simulink model "VOO_3K04"  (R2022a)
settings: Solver=FixedStepAuto  StartTime=0.0  StopTime=10.0  FixedStep=1e-3  RelTol=1e-3  EnableMultiTasking=on
undefined symbols (not defined in the file): D10, D11, D12, D2, D4, D5, D7, D8, D9, PTA0, PTA2, PTB23, PTB9, PTC3, PTC4, PTD0, PTD2, PTD3
libraries: frdmk64flib x11
settings Model: ExtModeTrigDuration=5  Creator=patri  LastModifiedBy=joshb
settings OptimizationCC: EnhancedBackFolding=on  PassReuseOutputArgsAs=Individual arguments  ZeroExternalMemoryAtStartup=off  ZeroInternalMemoryAtStartup=off  MaxStackSize=64  OptimizeBlockOrder=speed  DifferentSizesBufferReuse=on  OptimizationCustomize=off  EfficientTunableParamExpr=on
settings DebuggingCC: ParameterTunabilityLossMsg=error
settings HardwareCC: ProdBitPerPointer=32  ProdBitPerSizeT=32  ProdBitPerPtrDiffT=32  ProdLargestAtomicInteger=Long  ProdLargestAtomicFloat=Double  ProdWordSize=32  ProdHWDeviceType=ARM Compatible->ARM Cortex
settings SFSimCC: MATLABDynamicMemAlloc=off
settings RTWCC: SystemTargetFile=ert.tlc  HardwareBoard=NXP FRDM-K64F  TLCOptions="-aInlineSetEventsForThisBaseRateFcn=TLC_FALSE -aSuppressMultiTaskScheduler=TLC_FALSE  -aRateBasedStepFcn=0"  TemplateMakefile=ert_default_tmf  Toolchain=GNU Tools for ARM Embedded Processors
settings CodeAppCC: ForceParamTrailComments=on  IgnoreCustomStorageClasses=off  OperatorAnnotations=on  SimulinkDataObjDesc=on  SFDataObjDesc=on  InsertBlockDesc=on
settings ERTTargetCC: ExtModeTransport=4  ExtModeMexFile=sendToCommService

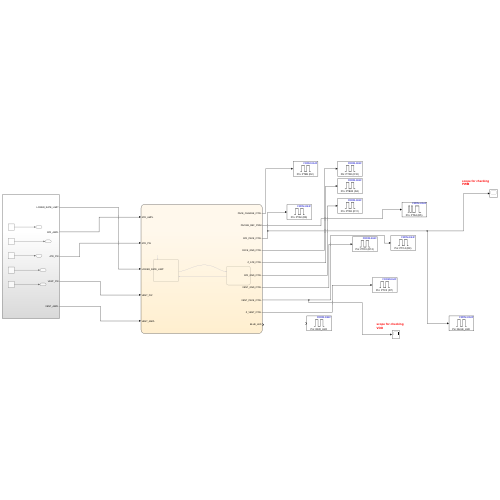
[thumbnail: Simulink's stored preview of the top-level diagram]
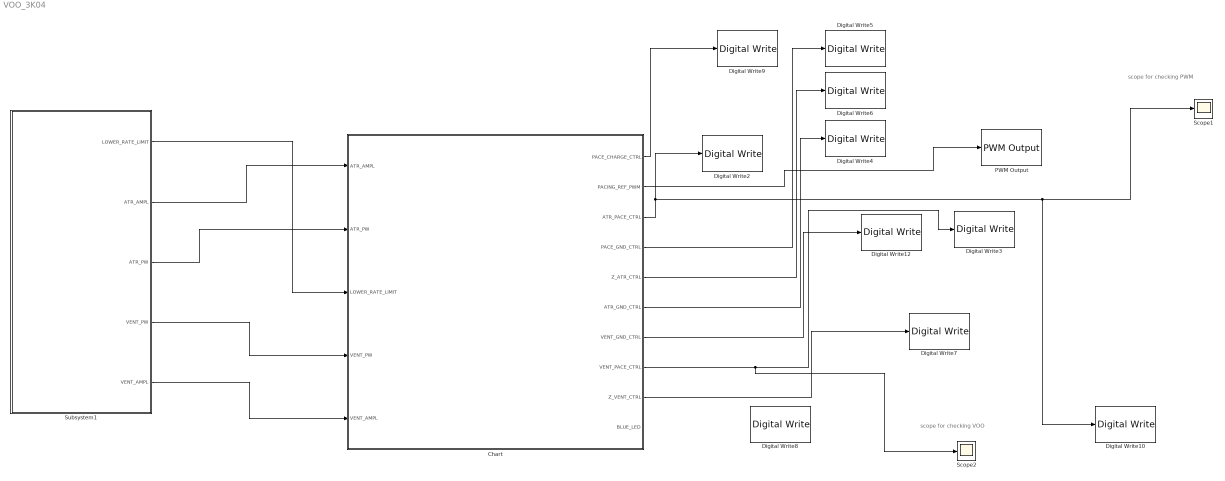
== system VOO_3K04 ==
  note: scope for checking PWM
  note: scope for checking VOO
  Chart : Stateflow chart  TreatAsAtomicUnit=on
  Digital Write10 : frdmk64flib/Digital Write  Whichpin=BLUE_LED
  Digital Write12 : frdmk64flib/Digital Write  Whichpin=PTD3 (D12)
  Digital Write2 : frdmk64flib/Digital Write  Whichpin=PTA0 (D8)
  Digital Write3 : frdmk64flib/Digital Write  Whichpin=PTC4 (D9)
  Digital Write4 : frdmk64flib/Digital Write  Whichpin=PTD2 (D11)
  Digital Write5 : frdmk64flib/Digital Write  Whichpin=PTD0 (D10)
  Digital Write6 : frdmk64flib/Digital Write  Whichpin=PTB23 (D4)
  Digital Write7 : frdmk64flib/Digital Write  Whichpin=PTC3 (D7)
  Digital Write8 : frdmk64flib/Digital Write  Whichpin=RED_LED
  Digital Write9 : frdmk64flib/Digital Write  Whichpin=PTB9 (D2)
  PWM Output : frdmk64flib/PWM Output  Whichpin=PTA2 (D5)  InitialFrequency=2000  InitialDutyCycle=0
  Scope1 : Scope
  Scope2 : Scope
  Subsystem1 : Subsystem
  wires:
  Chart/8(VENT_PACE_CTRL) -> Scope2/1, Digital Write3/1
  Chart/4(PACE_GND_CTRL) -> Digital Write5/1
  Chart/5(Z_ATR_CTRL) -> Digital Write6/1
  Chart/6(ATR_GND_CTRL) -> Digital Write4/1
  Chart/1(PACE_CHARGE_CTRL) -> Digital Write9/1
  Chart/7(VENT_GND_CTRL) -> Digital Write12/1
  Chart/9(Z_VENT_CTRL) -> Digital Write7/1
  Subsystem1/1(LOWER_RATE_LIMIT) -> Chart/3(LOWER_RATE_LIMIT)
  Subsystem1/3(ATR_PW) -> Chart/2(ATR_PW)
  Subsystem1/2(ATR_AMPL) -> Chart/1(ATR_AMPL)
  Chart/2(PACING_REF_PWM) -> PWM Output/1
  Chart/3(ATR_PACE_CTRL) -> Digital Write10/1, Scope1/1, Digital Write2/1
  Subsystem1/4(VENT_PW) -> Chart/4(VENT_PW)
  Subsystem1/5(VENT_AMPL) -> Chart/5(VENT_AMPL)

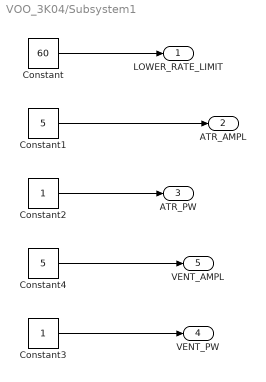
== system VOO_3K04/Subsystem1 ==
  Constant : Constant  Value=60
  Constant1 : Constant  Value=5
  Constant2 : Constant
  Constant3 : Constant
  Constant4 : Constant  Value=5
  LOWER_RATE_LIMIT : Outport
  ATR_AMPL : Outport  Port=2
  ATR_PW : Outport  Port=3
  VENT_PW : Outport  Port=4
  VENT_AMPL : Outport  Port=5
  wires:
  Constant/1 -> LOWER_RATE_LIMIT/1
  Constant1/1 -> ATR_AMPL/1
  Constant2/1 -> ATR_PW/1
  Constant4/1 -> VENT_AMPL/1
  Constant3/1 -> VENT_PW/1

== stateflow chart VOO_3K04/Chart ==
  state Charging_C23
    entry:
    VENT_PACE_CTRL = 0;
    VENT_GND_CTRL = 1;
    ATR_PACE_CTRL = 0;
    ATR_GND_CTRL = 0;
    PACE_GND_CTRL = 1;
    Z_VENT_CTRL = 0;
    Z_ATR_CTRL = 0;
    PACE_CHARGE_CTRL = 1;
    BLUE_LED = 0;
    PACING_REF_PWM = VENT_AMPL*10;
  state VENT_Pacing
    entry:
    PACE_CHARGE_CTRL = 0;
    VENT_PACE_CTRL = 1;
    VENT_GND_CTRL = 0;
    BLUE_LED = 1;
  (default) -> Charging_C23 : [1]
  Charging_C23 -> VENT_Pacing : [after(60000/(LOWER_RATE_LIMIT)- VENT_PW,msec)]
  VENT_Pacing -> Charging_C23 : [after(VENT_PW,msec)]
  data: PACE_CHARGE_CTRL output; PACING_REF_PWM output; ATR_PACE_CTRL output; PACE_GND_CTRL output; Z_ATR_CTRL output; ATR_GND_CTRL output; VENT_GND_CTRL output; VENT_PACE_CTRL output; Z_VENT_CTRL output; ATR_AMPL input; ATR_PW input; LOWER_RATE_LIMIT input; BLUE_LED output; VENT_PW input; VENT_AMPL input
